simulink model "Identificacao_Recursiva"  (R2013b)
settings: Solver=ode45  StartTime=0.0  StopTime=50  RelTol=1e-3
libraries: simulink x1
settings Model: Creator=Eduardo  LastModifiedBy=Eduardo

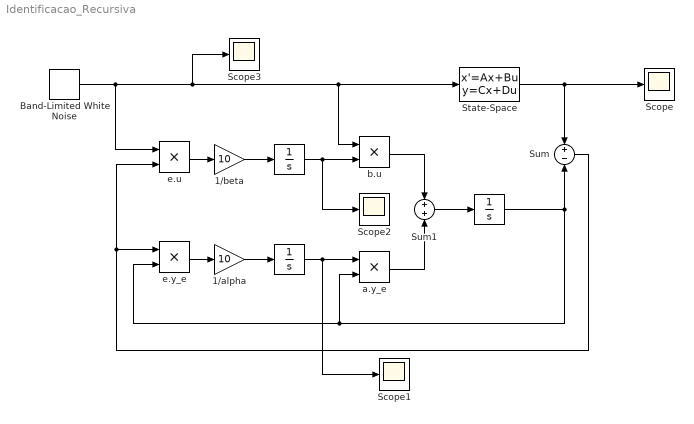
== system Identificacao_Recursiva ==
  " " : Integrator
  "  " : Integrator
  "   " : Integrator
  1/alpha : Gain  Gain=10
  1/beta : Gain  Gain=10
  Band-Limited White Noise : simulink/Sources/Band-Limited White Noise  Cov=[0.1]  Ts=0.1  seed=[23341]
  Scope{,1..3} (4 alike) : Scope
      Scope2 settings: SaveName=ScopeData2
      Scope3 settings: SaveName=ScopeData3
  State-Space : StateSpace  A=-1  D=0  X0=0
  Sum : Sum  Inputs=+|-
  Sum1 : Sum  Inputs=+|+
  a.y_e : Product
  b.u : Product
  e.u : Product
  e.y_e : Product
  wires:
  Band-Limited White Noise/1 -> e.u/1, Scope3/1, b.u/1, State-Space/1
  State-Space/1 -> Scope/1, Sum/1
  "   "/1 -> a.y_e/2, e.y_e/2, Sum/2
  Sum/1 -> e.u/2, e.y_e/1
  e.u/1 -> 1/beta/1
  e.y_e/1 -> 1/alpha/1
  1/beta/1 -> " "/1
  1/alpha/1 -> "  "/1
  " "/1 -> Scope2/1, b.u/2
  "  "/1 -> Scope1/1, a.y_e/1
  b.u/1 -> Sum1/1
  Sum1/1 -> "   "/1
  a.y_e/1 -> Sum1/2
